simulink model "prelab"  (R2022a)
settings: Solver=VariableStepAuto  StartTime=0.0  StopTime=2  FixedStep=1e-5  RelTol=1e-3
undefined symbols (not defined in the file or in its folder): A, Ad_hat_10, Ad_hat_100, Ad_hat_20, Ad_hat_50, B, Bd_hat_10, Bd_hat_100, Bd_hat_20, Bd_hat_50, K_d, K_d_10, K_d_20, K_d_50
settings Model: Creator=user  LastModifiedBy=user

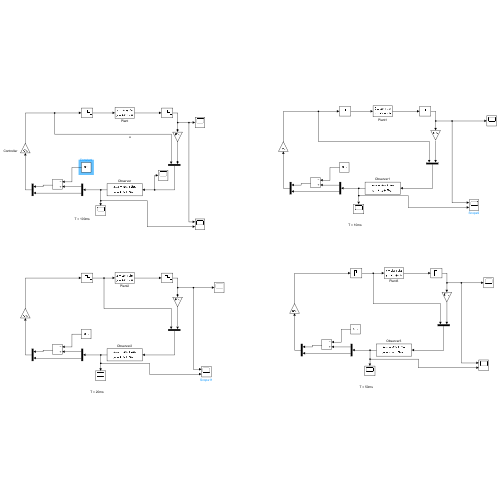
[thumbnail: Simulink's stored preview of the top-level diagram]
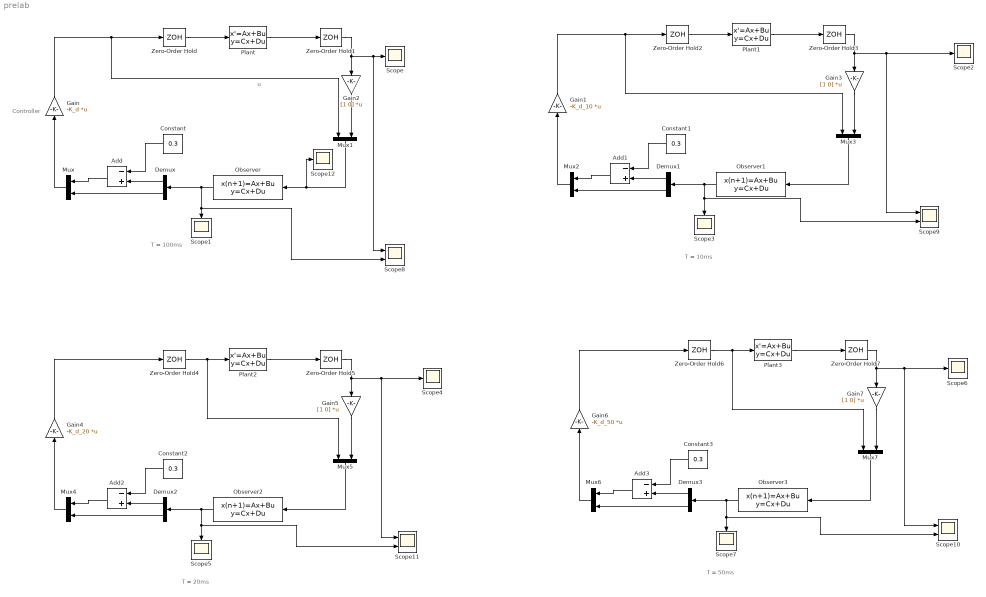
== system prelab ==
  note: Controller
  note: u
  note: T = 100ms
  note: T = 10ms
  note: T = 20ms
  note: T = 50ms
  Add{,1..3} (4 alike) : Sum  Inputs=-+
  Constant{,1..3} (4 alike) : Constant  Value=0.3
  Demux{,1..3} (4 alike) : Demux  Outputs=2
  Gain : Gain  Gain=-K_d  Multiplication=Matrix(K*u)
  Gain1 : Gain  Gain=-K_d_10  Multiplication=Matrix(K*u)
  Gain{2..3,5,7} (4 alike) : Gain  Gain=[1 0]  Multiplication=Matrix(K*u)
  Gain4 : Gain  Gain=-K_d_20  Multiplication=Matrix(K*u)
  Gain6 : Gain  Gain=-K_d_50  Multiplication=Matrix(K*u)
  Mux{,1..7} (8 alike) : Mux  Inputs=2
  Observer : DiscreteStateSpace  A=Ad_hat_100  B=Bd_hat_100  C=eye(2)  D=[0 0;0 0]  SampleTime=0.1
  Observer1 : DiscreteStateSpace  A=Ad_hat_10  B=Bd_hat_10  C=eye(2)  D=[0 0;0 0]  SampleTime=0.01
  Observer2 : DiscreteStateSpace  A=Ad_hat_20  B=Bd_hat_20  C=eye(2)  D=[0 0;0 0]  SampleTime=-1
  Observer3 : DiscreteStateSpace  A=Ad_hat_50  B=Bd_hat_50  C=eye(2)  D=[0 0;0 0]  SampleTime=-1
  Plant{,1..3} (4 alike) : StateSpace  A=A  B=B  C=eye(2)  D=[0;0]  InitialCondition=0
  Scope{,1..7,12} (9 alike) : Scope
  Scope{8..11} (4 alike) : Scope  NumInputPorts=2
  Zero-Order Hold : ZeroOrderHold  SampleTime=0.1
  Zero-Order Hold1 : ZeroOrderHold  SampleTime=0.1
  Zero-Order Hold2 : ZeroOrderHold  SampleTime=0.01
  Zero-Order Hold3 : ZeroOrderHold  SampleTime=0.01
  Zero-Order Hold4 : ZeroOrderHold  SampleTime=0.02
  Zero-Order Hold5 : ZeroOrderHold  SampleTime=0.02
  Zero-Order Hold6 : ZeroOrderHold  SampleTime=0.05
  Zero-Order Hold7 : ZeroOrderHold  SampleTime=0.05
  wires:
  Plant/1 -> Zero-Order Hold1/1
  Observer/1 -> Demux/1, Scope8/2, Scope1/1
  Demux/2 -> Mux/2
  Demux/1 -> Add/2
  Mux/1 -> Gain/1
  Add/1 -> Mux/1
  Gain/1 -> Mux1/1, Zero-Order Hold/1
  Constant/1 -> Add/1
  Zero-Order Hold/1 -> Plant/1
  Mux1/1 -> Scope12/1, Observer/1
  Gain2/1 -> Mux1/2
  Zero-Order Hold1/1 -> Scope8/1, Scope/1, Gain2/1
  Gain3/1 -> Mux3/2
  Zero-Order Hold2/1 -> Plant1/1
  Gain1/1 -> Mux3/1, Zero-Order Hold2/1
  Zero-Order Hold3/1 -> Scope9/1, Scope2/1, Gain3/1
  Demux1/1 -> Add1/2
  Plant1/1 -> Zero-Order Hold3/1
  Observer1/1 -> Demux1/1, Scope9/2, Scope3/1
  Constant1/1 -> Add1/1
  Demux1/2 -> Mux2/2
  Add1/1 -> Mux2/1
  Mux2/1 -> Gain1/1
  Mux3/1 -> Observer1/1
  Gain5/1 -> Mux5/2
  Zero-Order Hold4/1 -> Plant2/1, Mux5/1
  Gain4/1 -> Zero-Order Hold4/1
  Zero-Order Hold5/1 -> Scope11/1, Scope4/1, Gain5/1
  Demux2/1 -> Add2/2
  Plant2/1 -> Zero-Order Hold5/1
  Observer2/1 -> Demux2/1, Scope11/2, Scope5/1
  Constant2/1 -> Add2/1
  Demux2/2 -> Mux4/2
  Add2/1 -> Mux4/1
  Mux4/1 -> Gain4/1
  Mux5/1 -> Observer2/1
  Add3/1 -> Mux6/1
  Constant3/1 -> Add3/1
  Plant3/1 -> Zero-Order Hold7/1
  Observer3/1 -> Demux3/1, Scope10/2, Scope7/1
  Mux7/1 -> Observer3/1
  Demux3/2 -> Mux6/2
  Mux6/1 -> Gain6/1
  Zero-Order Hold7/1 -> Scope10/1, Scope6/1, Gain7/1
  Gain6/1 -> Zero-Order Hold6/1
  Zero-Order Hold6/1 -> Plant3/1, Mux7/1
  Gain7/1 -> Mux7/2
  Demux3/1 -> Add3/2
